simulink library "pcs_grc"  (R2024a)
settings: Solver=VariableStepAuto  StartTime=0.0  StopTime=10.0  RelTol=1e-3
undefined symbols (not defined in the file or in its folder): KPCS_bCurOffsVolVld_flg_ovrdflg, KPCS_bCurOffsVolVld_flg_ovrdval, KPCS_EnaSnsrSelfLrn_flg_ovrdflg, KPCS_EnaSnsrSelfLrn_flg_ovrdval, KPCS_MaxCurrReset_flg, KPCS_OffsFilCoeff_fac, KPCS_OffsFilTi_cnt, KPCS_PhaseCurSnsrVolDft_V, KPCS_PhaseCurSnsrVolVldMax_V, KPCS_PhaseCurSnsrVolVldMin_V, KPCS_UCurSnsr_Gain, KPCS_VCurSnsr_Gain, KPCS_WCurSnsr_Gain, PCS_iPaCSMor_C, PCS_iPaCSTrig_C, PCS_iPbCSMor_C, PCS_iPbCSTrig_C, PCS_iPcCSMor_C, PCS_iPcCSTrig_C, Spi1_f32_CurRng_C, Spi1_int32_CurOfsDl_C, SPI1_INT32_CUROFSDL_NULL, ZERO_FLOAT
libraries: Library x3
settings Model: Creator=FVT22063  LastModifiedBy=FVT22063

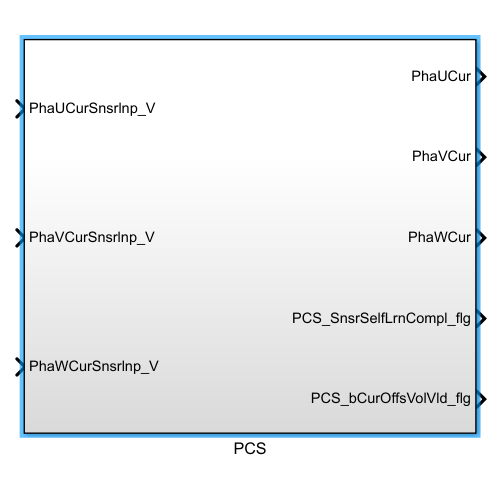
[thumbnail: Simulink's stored preview of the top-level diagram]
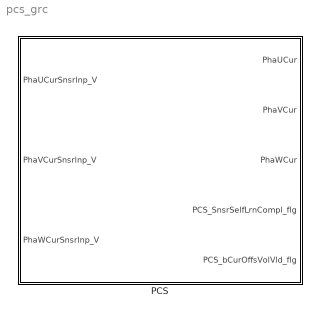
== system pcs_grc ==
  PCS : Subsystem

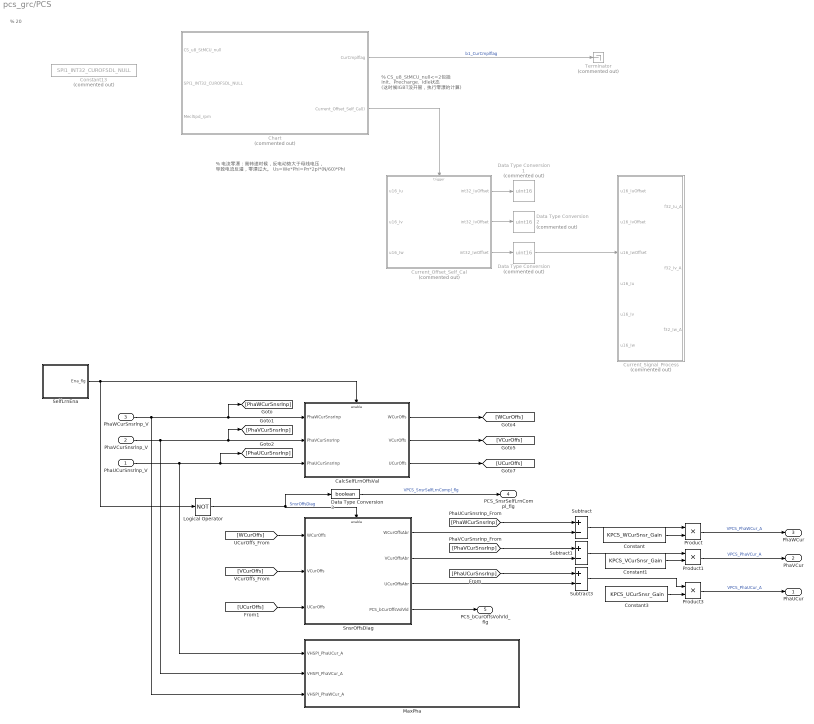
== system pcs_grc/PCS ==
  note: % 电流零漂：高转速时候，反电动势大于母线电压，
      | 导致电流反灌，零漂过大。
      | Us=We*Phi=Pn*2pi*(N/60)*Phi
  note: % 20
  note: % CS_u8_StMCU_null<=2包括
      | Init、Precharge、Idle状态
      | (这时候IGBT没开管，执行零漂的计算)
  PhaUCurSnsrlnp_V : Inport
  PhaVCurSnsrlnp_V : Inport  Port=2
  PhaWCurSnsrlnp_V : Inport  Port=3
  CalcSelfLrnOffsVal : Subsystem  TreatAsAtomicUnit=on
  Chart : Stateflow chart  Commented=on  TreatAsAtomicUnit=on
  Constant : Constant  Value=KPCS_WCurSnsr_Gain  OutDataTypeStr=single
  Constant1 : Constant  Value=KPCS_VCurSnsr_Gain  OutDataTypeStr=single
  Constant13 : Constant  Commented=on  Value=SPI1_INT32_CUROFSDL_NULL  OutDataTypeStr=int32
  Constant3 : Constant  Value=KPCS_UCurSnsr_Gain  OutDataTypeStr=single
  Current_Offset_Self_Cal : Subsystem  Commented=on  TreatAsAtomicUnit=on  RTWFcnName=Current_Offset_Self_Cal
      settings: RTWFcnNameOpts=User specified
  Current_Signal_Process : Subsystem  Commented=on
  Data Type Conversion : DataTypeConversion  Commented=on  OutDataTypeStr=uint16  SaturateOnIntegerOverflow=off  RndMeth=Floor
  Data Type Conversion1 : DataTypeConversion  Commented=on  OutDataTypeStr=uint16  SaturateOnIntegerOverflow=off  RndMeth=Floor
  Data Type Conversion2 : DataTypeConversion  Commented=on  OutDataTypeStr=uint16  SaturateOnIntegerOverflow=off  RndMeth=Floor
  Data Type Conversion3 : DataTypeConversion  OutDataTypeStr=boolean  SaturateOnIntegerOverflow=off  RndMeth=Floor
  Logical Operator : Logic  Operator=NOT  AllPortsSameDT=off  OutDataTypeStr=boolean
  MaxPha : Subsystem
  Product : Product  RndMeth=Zero
  Product1 : Product  RndMeth=Zero
  Product3 : Product  RndMeth=Zero
  SelfLrnEna : Subsystem
  SnsrOffsDiag : Subsystem
  Subtract : Sum  Inputs=+-
  Subtract1 : Sum  Inputs=+-
  Subtract3 : Sum  Inputs=+-
  Terminator : Terminator  Commented=on
  PhaUCur : Outport
  PhaVCur : Outport  Port=2
  PhaWCur : Outport  Port=3
  PCS_SnsrSelfLrnCompl_flg : Outport  Port=4
  PCS_bCurOffsVolVld_flg : Outport  Port=5
  wires:
  Chart/1(CurCmplflag) -> Terminator/1  "b1_CurCmplflag"
  Current_Offset_Self_Cal/1(int32_IuOffset) -> Data Type Conversion1/1
  Current_Offset_Self_Cal/2(int32_IvOffset) -> Data Type Conversion2/1
  Current_Offset_Self_Cal/3(int32_IwOffset) -> Data Type Conversion/1
  Data Type Conversion/1 -> Current_Signal_Process/3(u16_IwOffset)
  Chart/2(Current_Offset_Self_Cal()) -> Current_Offset_Self_Cal/Trigger
  SnsrOffsDiag/4(PCS_bCurOffsVolVld) -> PCS_bCurOffsVolVld_flg/1
  [PhaVCurSnsrInp] -> Subtract1/1
  [UCurOffs] -> SnsrOffsDiag/3(UCurOffs)
  CalcSelfLrnOffsVal/2(VCurOffs) -> [VCurOffs]
  [PhaUCurSnsrInp] -> Subtract3/1
  SnsrOffsDiag/3(UCurOffsAbr) -> Subtract3/2
  PhaVCurSnsrlnp_V/1 -> MaxPha/2(VHSPI_PhaVCur_A), CalcSelfLrnOffsVal/2(PhaVCurSnsrInp), [PhaVCurSnsrInp]
  SelfLrnEna/1(Ena_flg) -> CalcSelfLrnOffsVal/Enable, Logical Operator/1
  [WCurOffs] -> SnsrOffsDiag/1(WCurOffs)
  Product1/1 -> PhaVCur/1  "VPCS_PhaVCur_A"
  Data Type Conversion3/1 -> PCS_SnsrSelfLrnCompl_flg/1  "VPCS_SnsrSelfLrnCompl_flg"
  Constant/1 -> Product/2
  Subtract/1 -> Product/1
  [PhaWCurSnsrInp] -> Subtract/1
  Constant3/1 -> Product3/2
  Logical Operator/1 -> SnsrOffsDiag/Enable, Data Type Conversion3/1  "SnsrOffsDiag"
  Subtract3/1 -> Product3/1
  CalcSelfLrnOffsVal/3(UCurOffs) -> [UCurOffs]
  CalcSelfLrnOffsVal/1(WCurOffs) -> [WCurOffs]
  PhaUCurSnsrlnp_V/1 -> MaxPha/1(VHSPI_PhaUCur_A), [PhaUCurSnsrInp], CalcSelfLrnOffsVal/3(PhaUCurSnsrInp)
  Subtract1/1 -> Product1/1
  [VCurOffs] -> SnsrOffsDiag/2(VCurOffs)
  SnsrOffsDiag/1(WCurOffsAbr) -> Subtract/2
  PhaWCurSnsrlnp_V/1 -> MaxPha/3(VHSPI_PhaWCur_A), CalcSelfLrnOffsVal/1(PhaWCurSnsrInp), [PhaWCurSnsrInp]
  Product3/1 -> PhaUCur/1  "VPCS_PhaUCur_A"
  SnsrOffsDiag/2(VCurOffsAbr) -> Subtract1/2
  Constant1/1 -> Product1/2
  Product/1 -> PhaWCur/1  "VPCS_PhaWCur_A"

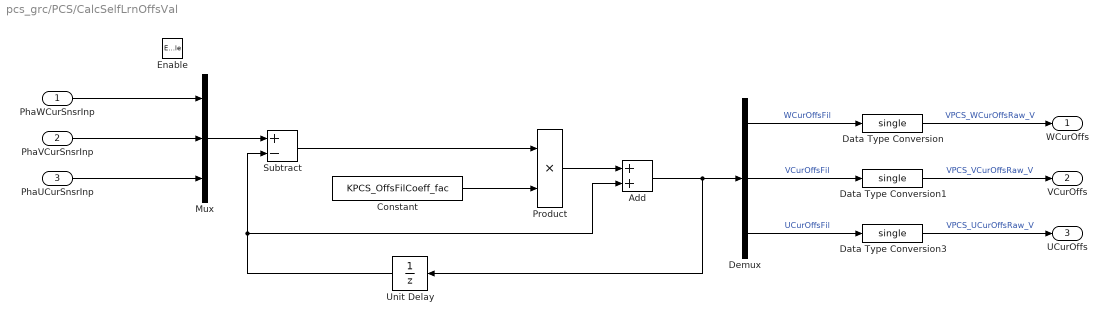
== system pcs_grc/PCS/CalcSelfLrnOffsVal ==
  PhaWCurSnsrInp : Inport
  PhaVCurSnsrInp : Inport  Port=2
  PhaUCurSnsrInp : Inport  Port=3
  Enable : EnablePort
  Add : Sum
  Constant : Constant  Value=KPCS_OffsFilCoeff_fac  OutDataTypeStr=single
  Data Type Conversion : DataTypeConversion  OutDataTypeStr=single  SaturateOnIntegerOverflow=off  RndMeth=Floor
  Data Type Conversion1 : DataTypeConversion  OutDataTypeStr=single  SaturateOnIntegerOverflow=off  RndMeth=Floor
  Data Type Conversion3 : DataTypeConversion  OutDataTypeStr=single  SaturateOnIntegerOverflow=off  RndMeth=Floor
  Demux : Demux  Outputs=3
  Mux : Mux  Inputs=3
  Product : Product  RndMeth=Zero
  Subtract : Sum  Inputs=+-
  Unit Delay : UnitDelay  SampleTime=-1
  WCurOffs : Outport
  VCurOffs : Outport  Port=2
  UCurOffs : Outport  Port=3
  wires:
  PhaWCurSnsrInp/1 -> Mux/1
  Unit Delay/1 -> Subtract/2, Add/2
  Subtract/1 -> Product/1
  Constant/1 -> Product/2
  Product/1 -> Add/1
  Add/1 -> Unit Delay/1, Demux/1
  Mux/1 -> Subtract/1
  PhaVCurSnsrInp/1 -> Mux/2
  Demux/1 -> Data Type Conversion/1  "WCurOffsFil"
  Demux/2 -> Data Type Conversion1/1  "VCurOffsFil"
  PhaUCurSnsrInp/1 -> Mux/3
  Demux/3 -> Data Type Conversion3/1  "UCurOffsFil"
  Data Type Conversion/1 -> WCurOffs/1  "VPCS_WCurOffsRaw_V"
  Data Type Conversion1/1 -> VCurOffs/1  "VPCS_VCurOffsRaw_V"
  Data Type Conversion3/1 -> UCurOffs/1  "VPCS_UCurOffsRaw_V"

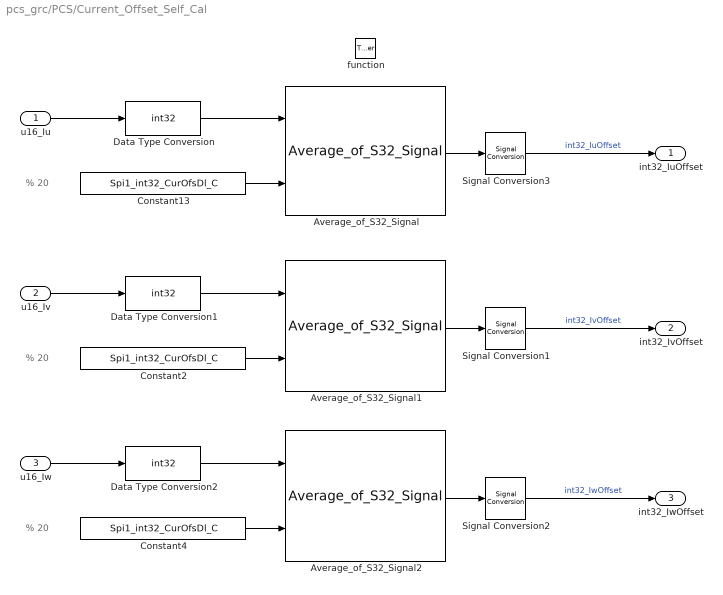
== system pcs_grc/PCS/Current_Offset_Self_Cal ==
  note: % 20
  note: % 20
  note: % 20
  u16_Iu : Inport  OutDataTypeStr=uint16
  u16_Iv : Inport  Port=2  OutDataTypeStr=uint16
  u16_Iw : Inport  Port=3  OutDataTypeStr=uint16
  function : TriggerPort  TriggerType=function-call  VariantControl=(inherit)
  Average_of_S32_Signal : Library/Average_of_S32_Signal
  Average_of_S32_Signal1 : Library/Average_of_S32_Signal
  Average_of_S32_Signal2 : Library/Average_of_S32_Signal
  Constant13 : Constant  Value=Spi1_int32_CurOfsDl_C  OutDataTypeStr=int32
  Constant2 : Constant  Value=Spi1_int32_CurOfsDl_C  OutDataTypeStr=int32
  Constant4 : Constant  Value=Spi1_int32_CurOfsDl_C  OutDataTypeStr=int32
  Data Type Conversion : DataTypeConversion  OutDataTypeStr=int32  SaturateOnIntegerOverflow=off  RndMeth=Floor
  Data Type Conversion1 : DataTypeConversion  OutDataTypeStr=int32  SaturateOnIntegerOverflow=off  RndMeth=Floor
  Data Type Conversion2 : DataTypeConversion  OutDataTypeStr=int32  SaturateOnIntegerOverflow=off  RndMeth=Floor
  Signal Conversion1 : SignalConversion  OverrideOpt=off
  Signal Conversion2 : SignalConversion  OverrideOpt=off
  Signal Conversion3 : SignalConversion  OverrideOpt=off
  int32_IuOffset : Outport  VectorParamsAs1DForOutWhenUnconnected=off
  int32_IvOffset : Outport  Port=2  VectorParamsAs1DForOutWhenUnconnected=off
  int32_IwOffset : Outport  Port=3  VectorParamsAs1DForOutWhenUnconnected=off
  wires:
  Constant13/1 -> Average_of_S32_Signal/2
  u16_Iu/1 -> Data Type Conversion/1
  Data Type Conversion/1 -> Average_of_S32_Signal/1
  Average_of_S32_Signal/1 -> Signal Conversion3/1
  Signal Conversion3/1 -> int32_IuOffset/1  "int32_IuOffset"
  Constant2/1 -> Average_of_S32_Signal1/2
  Average_of_S32_Signal1/1 -> Signal Conversion1/1
  Signal Conversion1/1 -> int32_IvOffset/1  "int32_IvOffset"
  Constant4/1 -> Average_of_S32_Signal2/2
  Average_of_S32_Signal2/1 -> Signal Conversion2/1
  Signal Conversion2/1 -> int32_IwOffset/1  "int32_IwOffset"
  Data Type Conversion1/1 -> Average_of_S32_Signal1/1
  u16_Iv/1 -> Data Type Conversion1/1
  Data Type Conversion2/1 -> Average_of_S32_Signal2/1
  u16_Iw/1 -> Data Type Conversion2/1

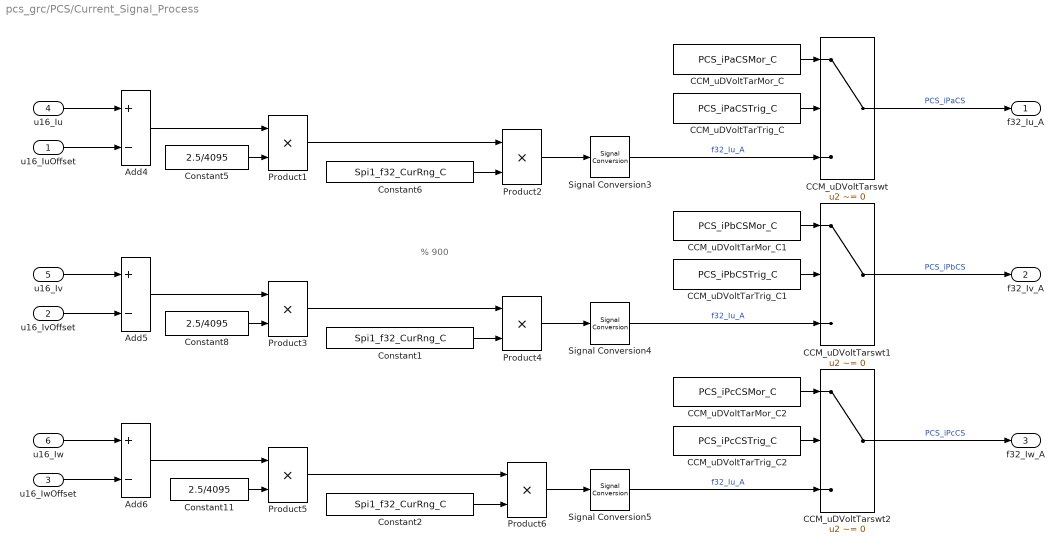
== system pcs_grc/PCS/Current_Signal_Process ==
  note: % 900
  u16_IuOffset : Inport  OutDataTypeStr=uint16
  u16_IvOffset : Inport  Port=2  OutDataTypeStr=uint16
  u16_IwOffset : Inport  Port=3  OutDataTypeStr=uint16
  u16_Iu : Inport  Port=4  OutDataTypeStr=uint16
  u16_Iv : Inport  Port=5  OutDataTypeStr=uint16
  u16_Iw : Inport  Port=6  OutDataTypeStr=uint16
  Add4 : Sum  Inputs=+-
  Add5 : Sum  Inputs=+-
  Add6 : Sum  Inputs=+-
  CCM_uDVoltTarMor_C : Constant  Value=PCS_iPaCSMor_C
  CCM_uDVoltTarMor_C1 : Constant  Value=PCS_iPbCSMor_C
  CCM_uDVoltTarMor_C2 : Constant  Value=PCS_iPcCSMor_C
  CCM_uDVoltTarTrig_C : Constant  Value=PCS_iPaCSTrig_C
  CCM_uDVoltTarTrig_C1 : Constant  Value=PCS_iPbCSTrig_C
  CCM_uDVoltTarTrig_C2 : Constant  Value=PCS_iPcCSTrig_C
  CCM_uDVoltTarswt : Switch  Criteria=u2 ~= 0  SaturateOnIntegerOverflow=off  InputSameDT=off
  CCM_uDVoltTarswt1 : Switch  Criteria=u2 ~= 0  SaturateOnIntegerOverflow=off  InputSameDT=off
  CCM_uDVoltTarswt2 : Switch  Criteria=u2 ~= 0  SaturateOnIntegerOverflow=off  InputSameDT=off
  Constant1 : Constant  Value=Spi1_f32_CurRng_C  OutDataTypeStr=single
  Constant11 : Constant  Value=2.5/4095  OutDataTypeStr=single
  Constant2 : Constant  Value=Spi1_f32_CurRng_C  OutDataTypeStr=single
  Constant5 : Constant  Value=2.5/4095  OutDataTypeStr=single
  Constant6 : Constant  Value=Spi1_f32_CurRng_C  OutDataTypeStr=single
  Constant8 : Constant  Value=2.5/4095  OutDataTypeStr=single
  Product{1..6} (6 alike) : Product
  Signal Conversion3 : SignalConversion  OverrideOpt=off
  Signal Conversion4 : SignalConversion  OverrideOpt=off
  Signal Conversion5 : SignalConversion  OverrideOpt=off
  f32_Iu_A : Outport  OutDataTypeStr=single  VectorParamsAs1DForOutWhenUnconnected=off
  f32_Iv_A : Outport  Port=2  OutDataTypeStr=single  VectorParamsAs1DForOutWhenUnconnected=off
  f32_Iw_A : Outport  Port=3  OutDataTypeStr=single  VectorParamsAs1DForOutWhenUnconnected=off
  wires:
  Constant5/1 -> Product1/2
  Add4/1 -> Product1/1
  Product1/1 -> Product2/1
  Constant6/1 -> Product2/2
  u16_Iv/1 -> Add5/1
  Constant8/1 -> Product3/2
  Product3/1 -> Product4/1
  Constant1/1 -> Product4/2
  Constant11/1 -> Product5/2
  Product5/1 -> Product6/1
  Constant2/1 -> Product6/2
  Product2/1 -> Signal Conversion3/1
  Product4/1 -> Signal Conversion4/1
  Product6/1 -> Signal Conversion5/1
  Signal Conversion3/1 -> CCM_uDVoltTarswt/3  "f32_Iu_A"
  u16_Iu/1 -> Add4/1
  u16_Iw/1 -> Add6/1
  Add5/1 -> Product3/1
  Add6/1 -> Product5/1
  u16_IuOffset/1 -> Add4/2
  u16_IvOffset/1 -> Add5/2
  u16_IwOffset/1 -> Add6/2
  CCM_uDVoltTarMor_C/1 -> CCM_uDVoltTarswt/1
  CCM_uDVoltTarTrig_C/1 -> CCM_uDVoltTarswt/2
  CCM_uDVoltTarswt/1 -> f32_Iu_A/1  "PCS_iPaCS"
  CCM_uDVoltTarTrig_C1/1 -> CCM_uDVoltTarswt1/2
  Signal Conversion4/1 -> CCM_uDVoltTarswt1/3  "f32_Iu_A"
  CCM_uDVoltTarswt1/1 -> f32_Iv_A/1  "PCS_iPbCS"
  CCM_uDVoltTarMor_C1/1 -> CCM_uDVoltTarswt1/1
  CCM_uDVoltTarTrig_C2/1 -> CCM_uDVoltTarswt2/2
  Signal Conversion5/1 -> CCM_uDVoltTarswt2/3  "f32_Iu_A"
  CCM_uDVoltTarswt2/1 -> f32_Iw_A/1  "PCS_iPcCS"
  CCM_uDVoltTarMor_C2/1 -> CCM_uDVoltTarswt2/1

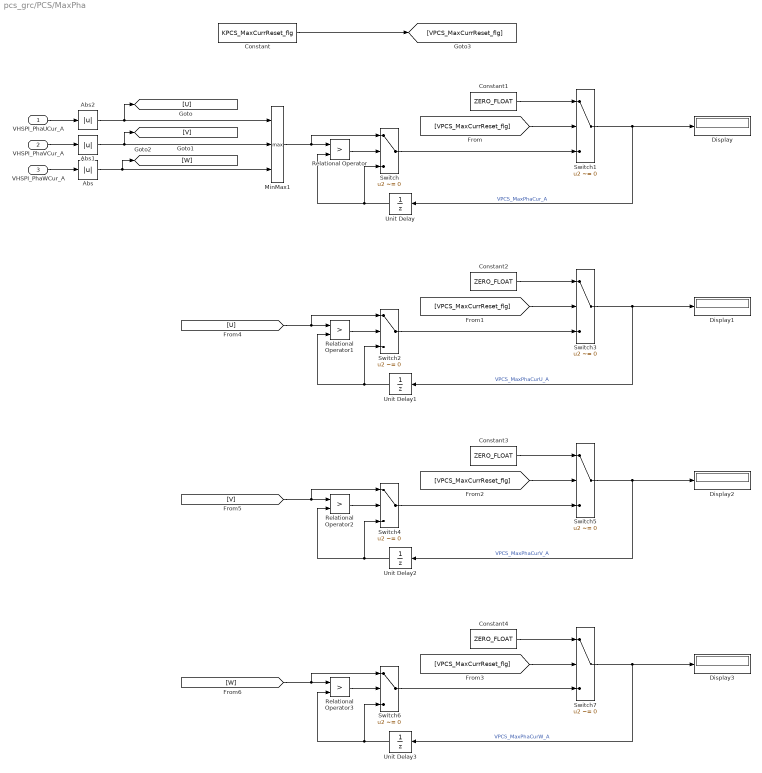
== system pcs_grc/PCS/MaxPha ==
  VHSPI_PhaUCur_A : Inport
  VHSPI_PhaVCur_A : Inport  Port=2
  VHSPI_PhaWCur_A : Inport  Port=3
  Abs : Abs  SaturateOnIntegerOverflow=off
  Abs1 : Abs  SaturateOnIntegerOverflow=off
  Abs2 : Abs  SaturateOnIntegerOverflow=off
  Constant : Constant  Value=KPCS_MaxCurrReset_flg
  Constant{1..4} (4 alike) : Constant  Value=ZERO_FLOAT
  Display{,1..3} (4 alike) : Display
  MinMax1 : MinMax  Function=max  Inputs=3
  Relational Operator{,1..3} (4 alike) : RelationalOperator  Operator=>  OutDataTypeStr=boolean  InputSameDT=off
  Switch{,1..7} (8 alike) : Switch  Criteria=u2 ~= 0  SaturateOnIntegerOverflow=off  InputSameDT=off
  Unit Delay{,1..3} (4 alike) : UnitDelay  SampleTime=-1
  wires:
  VHSPI_PhaVCur_A/1 -> Abs1/1
  MinMax1/1 -> Relational Operator/1, Switch/1
  Unit Delay/1 -> Relational Operator/2, Switch/3
  Abs1/1 -> [V], MinMax1/2
  Abs/1 -> [W], MinMax1/3
  Relational Operator/1 -> Switch/2
  VHSPI_PhaWCur_A/1 -> Abs/1
  VHSPI_PhaUCur_A/1 -> Abs2/1
  Abs2/1 -> MinMax1/1, [U]
  Switch/1 -> Switch1/3
  Switch1/1 -> Display/1, Unit Delay/1  "VPCS_MaxPhaCur_A"
  Constant1/1 -> Switch1/1
  Constant/1 -> [VPCS_MaxCurrReset_flg]
  [VPCS_MaxCurrReset_flg] -> Switch1/2
  [VPCS_MaxCurrReset_flg] -> Switch3/2
  Relational Operator1/1 -> Switch2/2
  Unit Delay1/1 -> Relational Operator1/2, Switch2/3
  [U] -> Relational Operator1/1, Switch2/1
  Switch3/1 -> Display1/1, Unit Delay1/1  "VPCS_MaxPhaCurU_A"
  Switch2/1 -> Switch3/3
  Constant2/1 -> Switch3/1
  [VPCS_MaxCurrReset_flg] -> Switch5/2
  Relational Operator2/1 -> Switch4/2
  Unit Delay2/1 -> Relational Operator2/2, Switch4/3
  [V] -> Relational Operator2/1, Switch4/1
  Switch5/1 -> Display2/1, Unit Delay2/1  "VPCS_MaxPhaCurV_A"
  Switch4/1 -> Switch5/3
  Constant3/1 -> Switch5/1
  [VPCS_MaxCurrReset_flg] -> Switch7/2
  Relational Operator3/1 -> Switch6/2
  Unit Delay3/1 -> Relational Operator3/2, Switch6/3
  [W] -> Relational Operator3/1, Switch6/1
  Switch7/1 -> Display3/1, Unit Delay3/1  "VPCS_MaxPhaCurW_A"
  Switch6/1 -> Switch7/3
  Constant4/1 -> Switch7/1

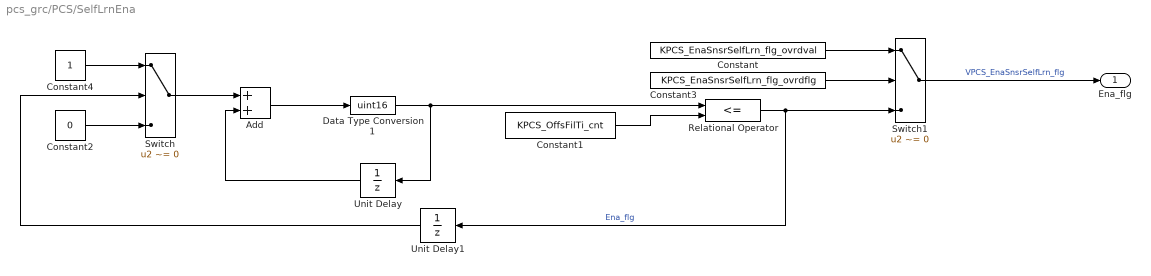
== system pcs_grc/PCS/SelfLrnEna ==
  Add : Sum
  Constant : Constant  Value=KPCS_EnaSnsrSelfLrn_flg_ovrdval
  Constant1 : Constant  Value=KPCS_OffsFilTi_cnt
  Constant2 : Constant  Value=0  OutDataTypeStr=uint16
  Constant3 : Constant  Value=KPCS_EnaSnsrSelfLrn_flg_ovrdflg
  Constant4 : Constant  OutDataTypeStr=uint16
  Data Type Conversion1 : DataTypeConversion  OutDataTypeStr=uint16  SaturateOnIntegerOverflow=off  RndMeth=Floor
  Relational Operator : RelationalOperator  Operator=<=  OutDataTypeStr=boolean  InputSameDT=off
  Switch : Switch  Criteria=u2 ~= 0  SaturateOnIntegerOverflow=off  InputSameDT=off
  Switch1 : Switch  Criteria=u2 ~= 0  SaturateOnIntegerOverflow=off  InputSameDT=off
  Unit Delay : UnitDelay  SampleTime=-1
  Unit Delay1 : UnitDelay  SampleTime=-1
  Ena_flg : Outport
  wires:
  Add/1 -> Data Type Conversion1/1
  Constant1/1 -> Relational Operator/2
  Relational Operator/1 -> Unit Delay1/1, Switch1/3  "Ena_flg"
  Data Type Conversion1/1 -> Unit Delay/1, Relational Operator/1
  Constant2/1 -> Switch/3
  Unit Delay1/1 -> Switch/2
  Unit Delay/1 -> Add/2
  Switch/1 -> Add/1
  Constant4/1 -> Switch/1
  Switch1/1 -> Ena_flg/1  "VPCS_EnaSnsrSelfLrn_flg"
  Constant3/1 -> Switch1/2
  Constant/1 -> Switch1/1

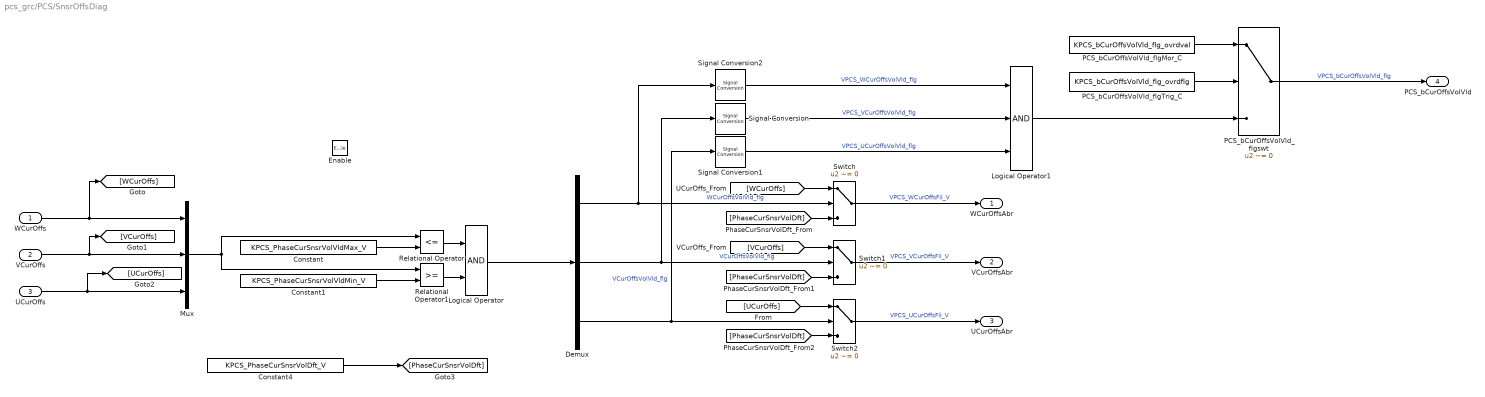
== system pcs_grc/PCS/SnsrOffsDiag ==
  WCurOffs : Inport
  VCurOffs : Inport  Port=2
  UCurOffs : Inport  Port=3
  Enable : EnablePort
  Constant : Constant  Value=KPCS_PhaseCurSnsrVolVldMax_V
  Constant1 : Constant  Value=KPCS_PhaseCurSnsrVolVldMin_V
  Constant4 : Constant  Value=KPCS_PhaseCurSnsrVolDft_V
  Demux : Demux  Outputs=3
  Logical Operator : Logic  AllPortsSameDT=off  OutDataTypeStr=boolean
  Logical Operator1 : Logic  Inputs=3  AllPortsSameDT=off  OutDataTypeStr=boolean
  Mux : Mux  Inputs=3
  PCS_bCurOffsVolVld_flgMor_C : Constant  Value=KPCS_bCurOffsVolVld_flg_ovrdval
  PCS_bCurOffsVolVld_flgTrig_C : Constant  Value=KPCS_bCurOffsVolVld_flg_ovrdflg
  PCS_bCurOffsVolVld_flgswt : Switch  Criteria=u2 ~= 0  SaturateOnIntegerOverflow=off  InputSameDT=off
  Relational Operator : RelationalOperator  Operator=<=  OutDataTypeStr=boolean  InputSameDT=off
  Relational Operator1 : RelationalOperator  OutDataTypeStr=boolean  InputSameDT=off
  Signal Conversion : SignalConversion  OverrideOpt=off
  Signal Conversion1 : SignalConversion  OverrideOpt=off
  Signal Conversion2 : SignalConversion  OverrideOpt=off
  Switch : Switch  Criteria=u2 ~= 0  SaturateOnIntegerOverflow=off  InputSameDT=off
  Switch1 : Switch  Criteria=u2 ~= 0  SaturateOnIntegerOverflow=off  InputSameDT=off
  Switch2 : Switch  Criteria=u2 ~= 0  SaturateOnIntegerOverflow=off  InputSameDT=off
  WCurOffsAbr : Outport
  VCurOffsAbr : Outport  Port=2
  UCurOffsAbr : Outport  Port=3
  PCS_bCurOffsVolVld : Outport  Port=4
  wires:
  Constant/1 -> Relational Operator/2
  WCurOffs/1 -> [WCurOffs], Mux/1
  VCurOffs/1 -> [VCurOffs], Mux/2
  Mux/1 -> Relational Operator/1, Relational Operator1/1
  Constant1/1 -> Relational Operator1/2
  Relational Operator/1 -> Logical Operator/1
  Relational Operator1/1 -> Logical Operator/2
  Logical Operator/1 -> Demux/1
  Demux/1 -> Signal Conversion2/1, Switch/2  "WCurOffsVolVld_flg"
  Switch/1 -> WCurOffsAbr/1  "VPCS_WCurOffsFil_V"
  [WCurOffs] -> Switch/1
  Demux/2 -> Signal Conversion/1, Switch1/2  "VCurOffsVolVld_flg"
  [VCurOffs] -> Switch1/1
  Constant4/1 -> [PhaseCurSnsrVolDft]
  [PhaseCurSnsrVolDft] -> Switch/3
  [PhaseCurSnsrVolDft] -> Switch1/3
  Switch1/1 -> VCurOffsAbr/1  "VPCS_VCurOffsFil_V"
  UCurOffs/1 -> [UCurOffs], Mux/3
  Switch2/1 -> UCurOffsAbr/1  "VPCS_UCurOffsFil_V"
  [PhaseCurSnsrVolDft] -> Switch2/3
  [UCurOffs] -> Switch2/1
  Demux/3 -> Signal Conversion1/1, Switch2/2  "VCurOffsVolVld_flg"
  Signal Conversion1/1 -> Logical Operator1/3  "VPCS_UCurOffsVolVld_flg"
  Signal Conversion/1 -> Logical Operator1/2  "VPCS_VCurOffsVolVld_flg"
  Signal Conversion2/1 -> Logical Operator1/1  "VPCS_WCurOffsVolVld_flg"
  PCS_bCurOffsVolVld_flgswt/1 -> PCS_bCurOffsVolVld/1  "VPCS_bCurOffsVolVld_flg"
  PCS_bCurOffsVolVld_flgMor_C/1 -> PCS_bCurOffsVolVld_flgswt/1
  PCS_bCurOffsVolVld_flgTrig_C/1 -> PCS_bCurOffsVolVld_flgswt/2
  Logical Operator1/1 -> PCS_bCurOffsVolVld_flgswt/3

== stateflow chart pcs_grc/PCS/Chart ==
  note: %CS_u8_StMCU_null<=2包括Init、Precharge、Idle状态
      | (这时候IGBT没开管，关波状态下，执行零漂的计算)
  note: %电机转速小于某转速，没有电流反灌，执行诊断
  note: %电流零漂计算到达字长
  (default) -> (junction 10)
  (junction 10) -> (junction 11) [order 1] : [(CS_u8_StMCU_null<=2)&&(MeclSpd_rpm<=800)]
  (junction 10) -> (junction 12) [order 2] : {
      | i=0;
      | }
  (junction 11) -> (junction 13) : {
      | Current_Offset_Self_Cal;
      | i++;
      | }
  (junction 13) -> (junction 16) [order 1] : [i>=SPI1_INT32_CUROFSDL_NULL]
  (junction 13) -> (junction 14) [order 2] : {
      | CurCmplflag=0;
      | }
  (junction 16) -> (junction 15) : {
      | CurCmplflag=1;%电流零漂校准完成
      | }
  (junction 14) -> (junction 12)
  (junction 15) -> (junction 14)
  (junction 12) -> (junction 25)
  data: CS_u8_StMCU_null input uint8; SPI1_INT32_CUROFSDL_NULL input int32; CurCmplflag output boolean; i local int32 =0; MeclSpd_rpm input single
  events: Current_Offset_Self_Cal output FUNCTION_CALL_EVENT
